simulink model "LLC_CMC_model"  (Simulink 7.1)
settings: Solver=ode5  StartTime=0.0  StopTime=0.2  FixedStep=2e-8  MaxStep=5e-8  MinStep=2.5e-8  RelTol=1e-15  AbsTol=1e-15
undefined symbols (not defined in the file or in its folder): DiscIntNeverNeededParam
libraries: simulink x3
settings Model: Creator=I14742  LastModifiedBy=I14742
settings SolverCC: InitialStep=2.5e-8  ExtrapolationOrder=2  NumberNewtonIterations=2  MaxConsecutiveMinStep=100  ShapePreserveControl=EnableAll

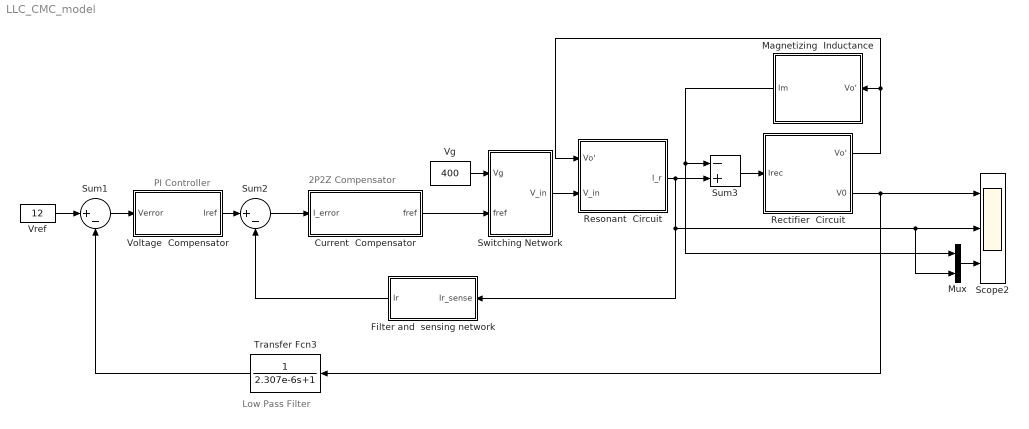
== system LLC_CMC_model ==
  note: PI Controller
  note: 2P2Z
      |  Compensator
  note: Low Pass
      |  Filter
  Current  Compensator : Subsystem
  Filter and  sensing network : Subsystem  Orientation=left
  Magnetizing  Inductance : Subsystem  Orientation=left
  Mux : Mux  Inputs=2
  Rectifier  Circuit : Subsystem
  Resonant  Circuit : Subsystem
  Scope2 : Scope  NumInputPorts=3
      settings: TimeRange=0.008064516129032261  YMin=11.78~-2.5~-1.25  YMax=11.95~2.5~1.25  MaxDataPoints=300000
  Sum1 : Sum  Inputs=|+-  OutDataType=sfix(16)  OutScaling=2^0
  Sum2 : Sum  Inputs=|+-  OutDataType=sfix(16)  OutScaling=2^0
  Sum3 : Sum  Inputs=-+  OutDataType=sfix(16)  OutScaling=2^0
  Switching Network : Subsystem
  Transfer Fcn3 : TransferFcn  Orientation=left  Numerator=1  Denominator=[2.307e-6 1]
  Vg : Constant  Value=400  OutDataType=sfix(16)  OutScaling=2^0
  Voltage  Compensator : Subsystem
  Vref : Constant  Value=12  OutDataType=sfix(16)  OutScaling=2^0
  wires:
  Sum3/1 -> Rectifier  Circuit/1(Irec)
  Vg/1 -> Switching Network/1(Vg)
  Switching Network/1(V_in) -> Resonant  Circuit/2(V_in)
  Resonant  Circuit/1(I_r) -> Sum3/2, Filter and  sensing network/1(Ir_sense), Scope2/2, Mux/2
  Magnetizing  Inductance/1(Im) -> Sum3/1, Mux/1
  Sum1/1 -> Voltage  Compensator/1(Verror)
  Vref/1 -> Sum1/1
  Transfer Fcn3/1 -> Sum1/2
  Mux/1 -> Scope2/3
  Voltage  Compensator/1(Iref) -> Sum2/1
  Filter and  sensing network/1(Ir) -> Sum2/2
  Sum2/1 -> Current  Compensator/1(I_error)
  Current  Compensator/1(fref) -> Switching Network/2(fref)
  Rectifier  Circuit/2(V0) -> Transfer Fcn3/1, Scope2/1
  Rectifier  Circuit/1(Vo') -> Resonant  Circuit/1(Vo'), Magnetizing  Inductance/1(Vo')

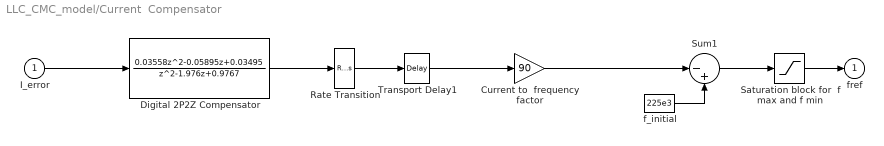
== system LLC_CMC_model/Current  Compensator ==
  I_error : Inport  OutDataType=sfix(16)  OutScaling=2^0
  Current to  frequency factor : Gain  Gain=90  ParameterDataType=sfix(16)  ParameterScaling=2^0  OutDataType=sfix(16)  OutScaling=2^0
  Digital 2P2Z Compensator : DiscreteTransferFcn  Numerator="[0.03558 -0.05895  0.03495]"  Denominator="[1 -1.976  0.9767]"  SampleTime=1/50e3
  Rate Transition : RateTransition  OutPortSampleTime=2e-8
  Saturation block for  f max and f min : Saturate  UpperLimit=300e3  LowerLimit=145e3  ZeroCross=off  OutDataType=sfix(16)  OutScaling=2^0
  Sum1 : Sum  Inputs=|-+  OutDataType=sfix(16)  OutScaling=2^0  SaturateOnIntegerOverflow=on  InputSameDT=on  OutDataTypeStr=Inherit: Same as first input
  Transport Delay1 : TransportDelay  DelayTime=2e-8
  f_initial : Constant  Value=225e3  OutDataType=sfix(16)  OutScaling=2^0  SampleTime=-1
  fref : Outport  OutDataType=sfix(16)  OutScaling=2^0  InitialOutput=0
  wires:
  f_initial/1 -> Sum1/2
  Sum1/1 -> Saturation block for  f max and f min/1
  Saturation block for  f max and f min/1 -> fref/1
  I_error/1 -> Digital 2P2Z Compensator/1
  Digital 2P2Z Compensator/1 -> Rate Transition/1
  Current to  frequency factor/1 -> Sum1/1
  Rate Transition/1 -> Transport Delay1/1
  Transport Delay1/1 -> Current to  frequency factor/1

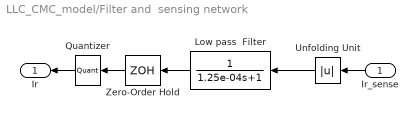
== system LLC_CMC_model/Filter and  sensing network ==
  Ir_sense : Inport  Orientation=left
  Low pass  Filter : TransferFcn  Orientation=left  Numerator=1  Denominator=[1.25e-04 1]
  Quantizer : Quantizer  Orientation=left  QuantizationInterval=1/1024  SampleTime=1/50e3
  Unfolding Unit : Abs  Orientation=left  ZeroCross=off  OutDataType=sfix(16)  OutScaling=2^0
  Zero-Order Hold : ZeroOrderHold  Orientation=left  SampleTime=1/50e3
  Ir : Outport  Orientation=left
  wires:
  Unfolding Unit/1 -> Low pass  Filter/1
  Low pass  Filter/1 -> Zero-Order Hold/1
  Zero-Order Hold/1 -> Quantizer/1
  Quantizer/1 -> Ir/1
  Ir_sense/1 -> Unfolding Unit/1

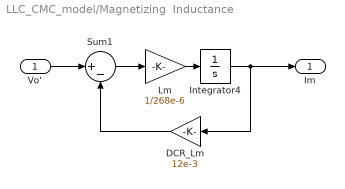
== system LLC_CMC_model/Magnetizing  Inductance ==
  Vo' : Inport
  DCR_Lm : Gain  Orientation=left  Gain=12e-3  ParameterDataType=sfix(16)  ParameterScaling=2^0  OutDataType=sfix(16)  OutScaling=2^0
  Integrator4 : Integrator  InitialCondition=-.68  UpperSaturationLimit=1.5  LowerSaturationLimit=-1.5
  Lm : Gain  Gain=1/268e-6  ParameterDataType=sfix(16)  ParameterScaling=2^0  OutDataType=sfix(16)  OutScaling=2^0
  Sum1 : Sum  Inputs=|+-  OutDataType=sfix(16)  OutScaling=2^0
  Im : Outport  OutDataType=sfix(16)  OutScaling=2^0
  wires:
  Lm/1 -> Integrator4/1
  Integrator4/1 -> DCR_Lm/1, Im/1
  Sum1/1 -> Lm/1
  DCR_Lm/1 -> Sum1/2
  Vo'/1 -> Sum1/1

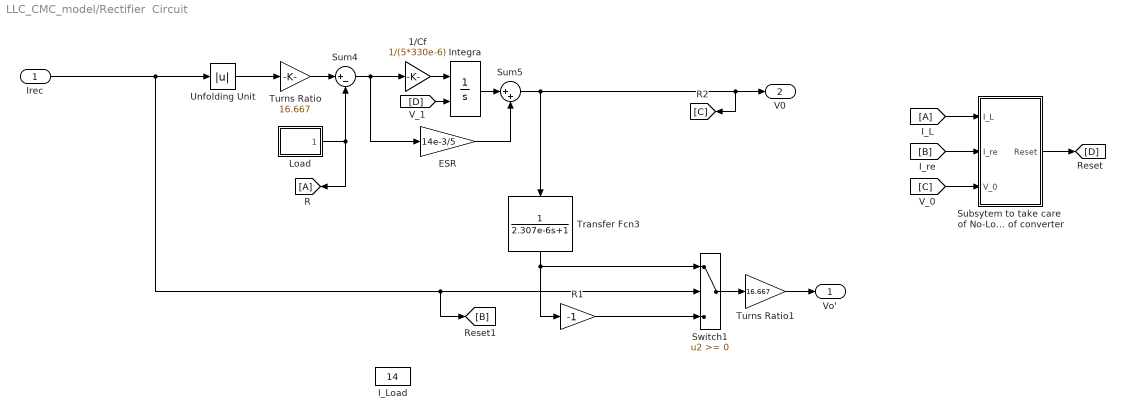
== system LLC_CMC_model/Rectifier  Circuit ==
  Irec : Inport  OutDataType=sfix(16)  OutScaling=2^0
  1/Cf : Gain  Gain=1/(5*330e-6)  ParameterDataType=sfix(16)  ParameterScaling=2^0  OutDataType=sfix(16)  OutScaling=2^0
  ESR : Gain  Gain=14e-3/5  ParameterDataType=sfix(16)  ParameterScaling=2^0  OutDataType=sfix(16)  OutScaling=2^0
  I_Load : Constant  Value=14  OutDataType=sfix(16)  OutScaling=2^0
  Integra : Integrator  ExternalReset=rising  InitialCondition=12  UpperSaturationLimit=122  LowerSaturationLimit=0
  Load : Subsystem
  R1 : Gain  Gain=-1  ParameterDataType=sfix(16)  ParameterScaling=2^0  OutDataType=sfix(16)  OutScaling=2^0
  Subsytem to take care  of No-Load operation of converter : Subsystem
  Sum4 : Sum  Inputs=|+-  OutDataType=sfix(16)  OutScaling=2^0
  Sum5 : Sum  Inputs=|++  OutDataType=sfix(16)  OutScaling=2^0
  Switch1 : Switch  OutDataType=sfix(16)  OutScaling=2^0  ZeroCross=off
  Transfer Fcn3 : TransferFcn  Orientation=down  Numerator=1  Denominator=[2.307e-6 1]
  Turns Ratio : Gain  Gain=16.667  ParameterDataType=sfix(16)  ParameterScaling=2^0  OutDataType=sfix(16)  OutScaling=2^0
  Turns Ratio1 : Gain  Gain=16.667  ParameterDataType=sfix(16)  ParameterScaling=2^0  OutDataType=sfix(16)  OutScaling=2^0
  Unfolding Unit : Abs  ZeroCross=off  OutDataType=sfix(16)  OutScaling=2^0
  Vo' : Outport  OutDataType=sfix(16)  OutScaling=2^0
  V0 : Outport  Port=2  OutDataType=sfix(16)  OutScaling=2^0
  wires:
  Irec/1 -> Unfolding Unit/1, Switch1/2, [B]
  Turns Ratio/1 -> Sum4/1
  Integra/1 -> Sum5/1
  Sum5/1 -> V0/1, [C], Transfer Fcn3/1
  ESR/1 -> Sum5/2
  1/Cf/1 -> Integra/1
  Switch1/1 -> Turns Ratio1/1
  R1/1 -> Switch1/3
  Unfolding Unit/1 -> Turns Ratio/1
  Turns Ratio1/1 -> Vo'/1
  Sum4/1 -> 1/Cf/1, ESR/1
  Load/1(I_Load) -> Sum4/2, [A]
  [A] -> Subsytem to take care  of No-Load operation of converter/1(I_L)
  [B] -> Subsytem to take care  of No-Load operation of converter/2(I_re)
  [C] -> Subsytem to take care  of No-Load operation of converter/3(V_0)
  Subsytem to take care  of No-Load operation of converter/1(Reset) -> [D]
  [D] -> Integra/2
  Transfer Fcn3/1 -> R1/1, Switch1/1

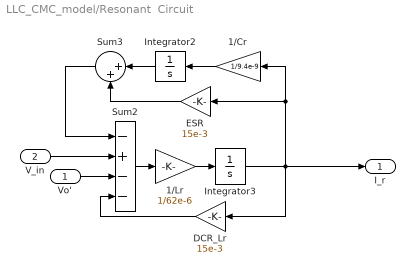
== system LLC_CMC_model/Resonant  Circuit ==
  Vo' : Inport
  V_in : Inport  Port=2
  1/Cr : Gain  Orientation=left  Gain=1/9.4e-9  ParameterDataType=sfix(16)  ParameterScaling=2^0  OutDataType=sfix(16)  OutScaling=2^0
  1/Lr : Gain  Gain=1/62e-6  ParameterDataType=sfix(16)  ParameterScaling=2^0  OutDataType=sfix(16)  OutScaling=2^0
  DCR_Lr : Gain  Orientation=left  Gain=15e-3  ParameterDataType=sfix(16)  ParameterScaling=2^0  OutDataType=sfix(16)  OutScaling=2^0
  ESR : Gain  Orientation=left  Gain=15e-3  ParameterDataType=sfix(16)  ParameterScaling=2^0  OutDataType=sfix(16)  OutScaling=2^0
  Integrator2 : Integrator  Orientation=left  InitialCondition=250  LimitOutput=on  UpperSaturationLimit=350  LowerSaturationLimit=50
  Integrator3 : Integrator  UpperSaturationLimit=100  LowerSaturationLimit=-100  IgnoreLimit=on
  Sum2 : Sum  Inputs=-+--  OutDataType=sfix(16)  OutScaling=2^0
  Sum3 : Sum  Orientation=left  Inputs=|++  OutDataType=sfix(16)  OutScaling=2^0
  I_r : Outport
  wires:
  1/Lr/1 -> Integrator3/1
  Sum2/1 -> 1/Lr/1
  Integrator3/1 -> DCR_Lr/1, 1/Cr/1, ESR/1, I_r/1
  1/Cr/1 -> Integrator2/1
  Vo'/1 -> Sum2/3
  V_in/1 -> Sum2/2
  DCR_Lr/1 -> Sum2/4
  Integrator2/1 -> Sum3/1
  Sum3/1 -> Sum2/1
  ESR/1 -> Sum3/2

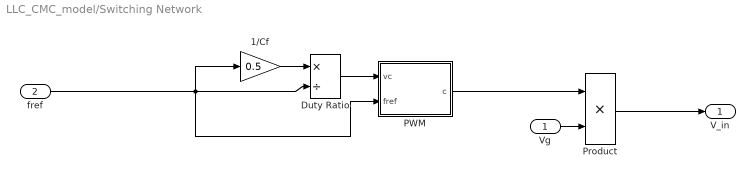
== system LLC_CMC_model/Switching Network ==
  Vg : Inport
  fref : Inport  Port=2
  1/Cf : Gain  Gain=0.5  ParameterDataType=sfix(16)  ParameterScaling=2^0  OutDataType=sfix(16)  OutScaling=2^0
  Duty Ratio : Product  Inputs=*/  OutDataType=sfix(16)  OutScaling=2^-10
  PWM : Subsystem
  Product : Product  OutDataType=sfix(16)  OutScaling=2^0  RndMeth=Zero
  V_in : Outport
  wires:
  PWM/1(c) -> Product/1
  Vg/1 -> Product/2
  Product/1 -> V_in/1
  1/Cf/1 -> Duty Ratio/1
  Duty Ratio/1 -> PWM/1(vc)
  fref/1 -> Duty Ratio/2, 1/Cf/1, PWM/2(fref)

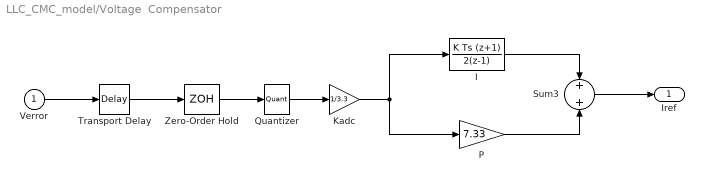
== system LLC_CMC_model/Voltage  Compensator ==
  Verror : Inport  OutDataType=sfix(16)  OutScaling=2^0
  I : DiscreteIntegrator  IntegratorMethod=Integration: Trapezoidal  gainval=25000  SampleTime=1/50000  OutDataType=sfix(16)  OutScaling=2^0  LimitOutput=on  UpperSaturationLimit=12  LowerSaturationLimit=-2  ICPrevOutput=DiscIntNeverNeededParam  ICPrevScaledInput=DiscIntNeverNeededParam
  Kadc : Gain  Gain=1/3.3  ParameterDataType=sfix(16)  ParameterScaling=2^0  OutDataType=sfix(16)  OutScaling=2^0
  P : Gain  Gain=7.33  ParameterDataType=sfix(16)  ParameterScaling=2^0  OutDataType=sfix(16)  OutScaling=2^0  SampleTime=1/50e3
  Quantizer : Quantizer  QuantizationInterval=1/1024  SampleTime=1/50e3
  Sum3 : Sum  Inputs=+|+  OutDataType=sfix(16)  OutScaling=2^0  SaturateOnIntegerOverflow=on  InputSameDT=on  OutDataTypeStr=Inherit: Same as first input
  Transport Delay : TransportDelay  DelayTime=2e-8
  Zero-Order Hold : ZeroOrderHold  SampleTime=1/50e3
  Iref : Outport
  wires:
  Quantizer/1 -> Kadc/1
  Verror/1 -> Transport Delay/1
  Zero-Order Hold/1 -> Quantizer/1
  Transport Delay/1 -> Zero-Order Hold/1
  Kadc/1 -> I/1, P/1
  Sum3/1 -> Iref/1
  P/1 -> Sum3/2
  I/1 -> Sum3/1

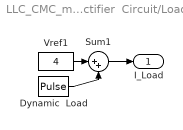
== system LLC_CMC_model/Rectifier  Circuit/Load ==
  Dynamic  Load : DiscretePulseGenerator  PulseType=Time based  Amplitude=8  Period=4e-3  PulseWidth=50  PhaseDelay=16e-3
  Sum1 : Sum  Inputs=|++  OutDataType=sfix(16)  OutScaling=2^0
  Vref1 : Constant  Value=4  OutDataType=sfix(16)  OutScaling=2^0
  I_Load : Outport  OutDataType=sfix(16)  OutScaling=2^0
  wires:
  Vref1/1 -> Sum1/1
  Dynamic  Load/1 -> Sum1/2
  Sum1/1 -> I_Load/1

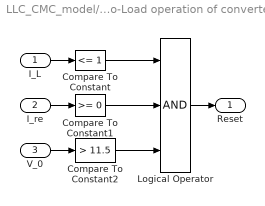
== system LLC_CMC_model/Rectifier  Circuit/Subsytem to take care  of No-Load operation of converter ==
  I_L : Inport
  I_re : Inport  Port=2
  V_0 : Inport  Port=3
  Compare To Constant : simulink/Logic and Bit Operations/Compare To Constant  SystemSampleTime=-1  relop=<=  const=1  LogicOutDataTypeMode=boolean  ZeroCross=off
  Compare To Constant1 : simulink/Logic and Bit Operations/Compare To Constant  SystemSampleTime=-1  relop=>=  const=0  LogicOutDataTypeMode=boolean  ZeroCross=off
  Compare To Constant2 : simulink/Logic and Bit Operations/Compare To Constant  SystemSampleTime=-1  relop=>  const=11.5  LogicOutDataTypeMode=boolean  ZeroCross=off
  Logical Operator : Logic  Inputs=3  AllPortsSameDT=off  OutDataTypeMode=boolean  OutDataTypeStr=boolean
  Reset : Outport
  wires:
  Compare To Constant/1 -> Logical Operator/1
  Compare To Constant1/1 -> Logical Operator/2
  Compare To Constant2/1 -> Logical Operator/3
  I_L/1 -> Compare To Constant/1
  I_re/1 -> Compare To Constant1/1
  Logical Operator/1 -> Reset/1
  V_0/1 -> Compare To Constant2/1

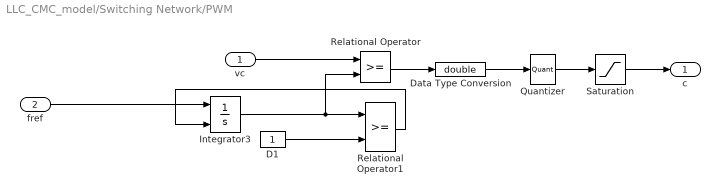
== system LLC_CMC_model/Switching Network/PWM ==
  vc : Inport  OutDataType=fixdt(1, 16)  OutScaling=2^0
  fref : Inport  Port=2  OutDataType=fixdt(1, 16)  OutScaling=2^0
  D1 : Constant  OutDataType=sfix(16)  OutScaling=2^0
  Data Type Conversion : DataTypeConversion  OutDataTypeMode=double  OutDataType=sfix(16)  OutScaling=2^0  OutDataTypeStr=double
  Integrator3 : Integrator  ExternalReset=rising  UpperSaturationLimit=100  LowerSaturationLimit=-100  IgnoreLimit=on
  Quantizer : Quantizer  QuantizationInterval=1/1024
  Relational Operator : RelationalOperator  LogicOutDataTypeMode=boolean  OutDataTypeStr=boolean
  Relational Operator1 : RelationalOperator  LogicOutDataTypeMode=boolean  OutDataTypeStr=boolean
  Saturation : Saturate  UpperLimit=1  LowerLimit=0  OutDataType=sfix(16)  OutScaling=2^0
  c : Outport  OutDataType=fixdt(1, 16)  OutScaling=2^0
  wires:
  vc/1 -> Relational Operator/1
  Relational Operator/1 -> Data Type Conversion/1
  Saturation/1 -> c/1
  Integrator3/1 -> Relational Operator1/1, Relational Operator/2
  D1/1 -> Relational Operator1/2
  Relational Operator1/1 -> Integrator3/2
  fref/1 -> Integrator3/1
  Data Type Conversion/1 -> Quantizer/1
  Quantizer/1 -> Saturation/1
